simulink model "Dynamic"  (R2021a)
settings: Solver=VariableStepAuto  StartTime=0.0  StopTime=10.0  RelTol=1e-3
settings Model: Creator=Araz  LastModifiedBy=Araz

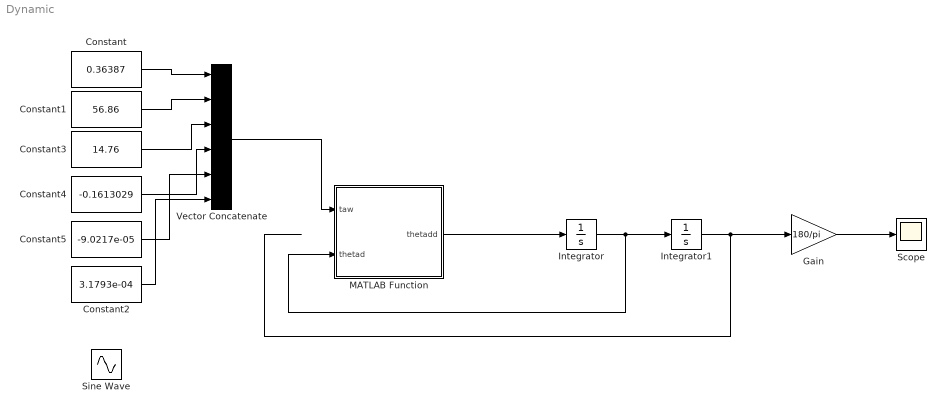
== system Dynamic ==
  Constant : Constant  Value=0.36387
  Constant1 : Constant  Value=56.86
  Constant2 : Constant  Value=3.1793e-04
  Constant3 : Constant  Value=14.76
  Constant4 : Constant  Value=-0.1613029
  Constant5 : Constant  Value=-9.0217e-05
  Gain : Gain  Gain=180/pi
  Integrator : Integrator
  Integrator1 : Integrator
  MATLAB Function : MATLAB Function  TreatAsAtomicUnit=on
  Scope : Scope
  Sine Wave : Sin  Frequency=2  SampleTime=0
  Vector Concatenate : Concatenate  NumInputs=6
  wires:
  MATLAB Function/1(thetadd) -> Integrator/1
  Integrator/1 -> MATLAB Function/2(thetad), Integrator1/1
  Integrator1/1 -> Gain/1
  Constant/1 -> Vector Concatenate/1
  Constant1/1 -> Vector Concatenate/2
  Constant3/1 -> Vector Concatenate/3
  Constant4/1 -> Vector Concatenate/4
  Constant5/1 -> Vector Concatenate/5
  Constant2/1 -> Vector Concatenate/6
  Vector Concatenate/1 -> MATLAB Function/1(taw)
  Gain/1 -> Scope/1

== matlab function Dynamic/MATLAB Function ==
  data: taw input; thetadd output; thetad input
function thetadd = fcn(taw,thetad)
M=[-0.514999084951298,0.139627040436924,0.00283580018469198,0.00499999999999812,-0.000649519052839942,0.00121201905283552;-1.77635683940025e-15,-2.31110214770077,-0.624510142736139,0,-0.00129903810567633,-0.000375000000000014;0,-0.185907897700785,-0.203220249999999,0,-0.00129903810567633,-0.000375000000000014;0.000832499999999944,0.00370095956307277,0.00567160036938424,0.0100000000000000,0,0.00129903810567666;0,0,0,0,0.00150000000000000,0;0,0,0,0,0,0.00150000000000000];
C=[-3.25422712372510,0.239189266414256,-0.00548766191766559,-0.0186441517773097,-0.000494150087808620,0;-0.490427844522568,-0.368580636409585,-0.573579418019513,-0.00368787844429974,-0.000804372410215803,0;0.819059318291849,0.555331731978775,-0.0709569423672987,-0.00212366888122251,-0.000804372410215803,0;0.00665062103159625,-0.000898701950552652,-0.000160052319936890,0.00273712499999999,-0.000396309255133898,0;-0.000890507160142345,-0.00207280333559595,-0.00207280333559595,-0.000306356486588745,0.000867500000000000,0;0.00126188317179060,-0.000663816662025630,-0.000663816662025630,0.00137156773324360,-0.000290118510267787,0];
G=[1.33226762955019e-15;57.2089881116302;14.6705473060650;-0.163336500000000;0;0];
thetadd=zeros(6,1);
thetadd=inv(M)*(taw- C*thetad - G);
